simulink model "sSpiegelPadStrom"  (R2012b)
settings: Solver=ode45  StartTime=0.0  StopTime=10.0  RelTol=1e-3
values from neighbouring files (symbols this model uses):
  J = 93.3e-9    (= 9.33e-08)    [msSpiegel.m]    (also in msSpiegel_PID.m; msSpiegel_Pad.m; msSpiegel_Pad_Neue_Werte.m = 9.33e-09; msSpiegel_Pad_Neue_Werte_Strom.m = 9.33e-10)
  KMPHI = 6.3e-2    (= 0.063)    [msSpiegel.m]    (also in msSpiegel_PID.m; msSpiegel_Pad.m; msSpiegel_Pad_Neue_Werte.m = 0.035; msSpiegel_Pad_Neue_Werte_Strom.m = 0.035)
  LA = RA*TA    (= 0.000448)    [msSpiegel.m]    (also in msSpiegel_PID.m; msSpiegel_Pad.m; msSpiegel_Pad_Neue_Werte.m = 3e-06; msSpiegel_Pad_Neue_Werte_Strom.m = 3e-06)
  Mspiegel = 130.25e-3    (= 0.13025)    [msSpiegel.m]    (also in msSpiegel_PID.m; msSpiegel_Pad.m; msSpiegel_Pad_Neue_Werte.m = 3.025e-05; msSpiegel_Pad_Neue_Werte_Strom.m = 3.025e-05)
  phi = 0.4    [Sensor_initieren.m]    (also in msSpiegel.m = 0.174532925199; msSpiegel_PID.m = 0.349065850399; msSpiegel_Pad.m = 0.349065850399; msSpiegel_Pad_Neue_Werte.m = 0.349065850399)
  r = []    [faltungsfunktionen.m]    (also in faltungsfunktionen3.m; msSpiegel.m = 6e-05; msSpiegel_PID.m = 6e-05; msSpiegel_Pad.m = 6e-05)
  RA = .16    (= 0.16)    [msSpiegel.m]    (also in msSpiegel_PID.m; msSpiegel_Pad.m; msSpiegel_Pad_Neue_Werte.m = 0.1; msSpiegel_Pad_Neue_Werte_Strom.m = 0.1)
settings Model: Creator=froriep  LastModifiedBy=michamann
settings DataIOCC: SignalLoggingSaveFormat=ModelDataLogs
settings DebuggingCC: FcnCallInpInsideContextMsg=EnableAllAsWarning
settings GRTTargetCC: CombineOutputUpdateFcns=off  GRTInterface=on

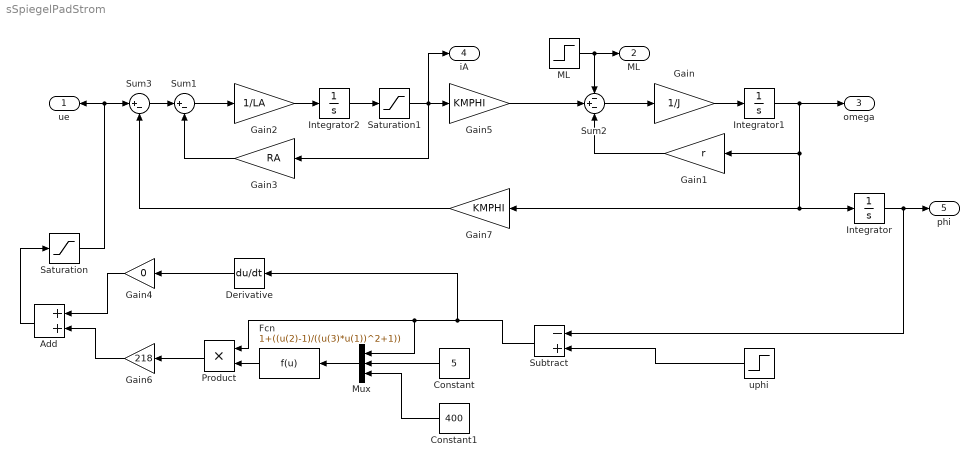
== system sSpiegelPadStrom ==
  Add : Sum
  Constant : Constant  Value=5
  Constant1 : Constant  Value=400
  Derivative : Derivative
  Fcn : Fcn  Expr=1+((u(2)-1)/((u(3)*u(1))^2+1))
  Gain : Gain  Gain=1/J
  Gain1 : Gain  Gain=r
  Gain2 : Gain  Gain=1/LA
  Gain3 : Gain  Gain=RA
  Gain4 : Gain  Gain=0
  Gain5 : Gain  Gain=KMPHI
  Gain6 : Gain  Gain=218
  Gain7 : Gain  Gain=KMPHI
  Integrator : Integrator
  Integrator1 : Integrator
  Integrator2 : Integrator
  ML : Step  Time=0  After=Mspiegel  SampleTime=0
  Mux : Mux  Inputs=3
  Product : Product  RndMeth=Zero
  Saturation : Saturate  UpperLimit=24  LowerLimit=-24
  Saturation1 : Saturate  UpperLimit=10  LowerLimit=-10
  Subtract : Sum  Inputs=-+  AccumDataTypeStr=double  OutDataTypeStr=double
  Sum1 : Sum  Inputs=|+-
  Sum2 : Sum  Inputs=-+-
  Sum3 : Sum  Inputs=|+-
  uphi : Step  Time=100  Before=phi  After=phi  SampleTime=0
  "ue " : Outport
  "ML " : Outport  Port=2
  omega : Outport  Port=3
  iA : Outport  Port=4
  phi : Outport  Port=5
  wires:
  Integrator1/1 -> Integrator/1, Gain7/1, Gain1/1, omega/1
  Gain/1 -> Integrator1/1
  Sum2/1 -> Gain/1
  Gain1/1 -> Sum2/3
  Gain2/1 -> Integrator2/1
  Sum1/1 -> Gain2/1
  Gain5/1 -> Sum2/2
  ML/1 -> Sum2/1, "ML "/1
  Sum3/1 -> Sum1/1
  Gain3/1 -> Sum1/2
  Gain7/1 -> Sum3/2
  Integrator/1 -> Subtract/1, phi/1
  uphi/1 -> Subtract/2
  Subtract/1 -> Derivative/1, Mux/1, Product/1
  Product/1 -> Gain6/1
  Gain6/1 -> Add/2
  Derivative/1 -> Gain4/1
  Gain4/1 -> Add/1
  Fcn/1 -> Product/2
  Mux/1 -> Fcn/1
  Constant/1 -> Mux/2
  Constant1/1 -> Mux/3
  Add/1 -> Saturation/1
  Saturation/1 -> "ue "/1, Sum3/1
  Integrator2/1 -> Saturation1/1
  Saturation1/1 -> Gain3/1, iA/1, Gain5/1
